simulink model "Plant_With_Time_Delay"  (R2023b)
settings: Solver=VariableStepAuto  StartTime=0.0  StopTime=20  RelTol=1e-3
settings Model: Creator=senpa  LastModifiedBy=acer

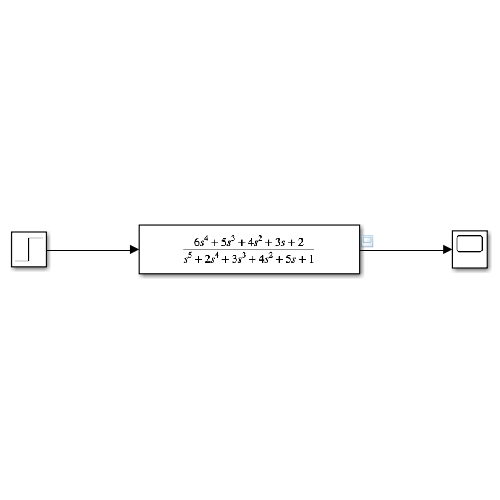
[thumbnail: Simulink's stored preview of the top-level diagram]
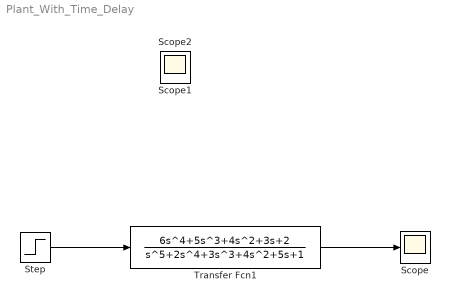
== system Plant_With_Time_Delay ==
  Scope : Scope
  Step : Step  Time=0.1  SampleTime=0
  Transfer Fcn1 : TransferFcn  Numerator=[6,5,4,3,2]  Denominator=[1,2,3,4,5,1]
  Scope1 : Scope
  Scope2 : Scope
  wires:
  Transfer Fcn1/1 -> Scope/1
  Step/1 -> Transfer Fcn1/1
